simulink model "Vending_Machine"  (R2020b)
settings: Solver=VariableStepAuto  StartTime=0.0  StopTime=10.0  RelTol=1e-3
settings Model: Creator=shubham sharma  LastModifiedBy=shubham sharma

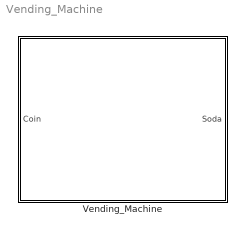
== system Vending_Machine ==
  Vending_Machine : Stateflow chart  TreatAsAtomicUnit=on

== stateflow chart Vending_Machine/Vending_Machine ==
  settings: stateMachineType=MEALY_MACHINE  initializeOutput=1
  state Dime_In
  state No_cash
  state Nickel_In
  No_cash -> Dime_In [order 2] : [Coin==2]{Soda=0}
  Dime_In -> No_cash [order 1] : [Coin==1]{Soda=1}
  Dime_In -> Nickel_In [order 2] : [Coin==2]{Soda=1}
  Nickel_In -> Dime_In [order 1] : [Coin==1]{Soda=0}
  No_cash -> Nickel_In [order 1] : [Coin==1]{Soda=0}
  (default) -> No_cash
  Nickel_In -> No_cash [order 2] : [Coin==2]{Soda=1}
  data: Coin input; Soda output double
